simulink model "polyforest2"  (R2024a)
settings: Solver=VariableStepAuto  StartTime=0.0  StopTime=60  RelTol=1e-3
libraries: vrlib x1
settings Model: Creator=samoe  LastModifiedBy=samoe

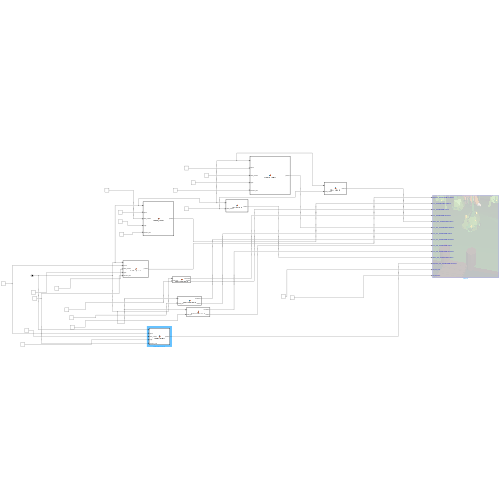
[thumbnail: Simulink's stored preview of the top-level diagram]
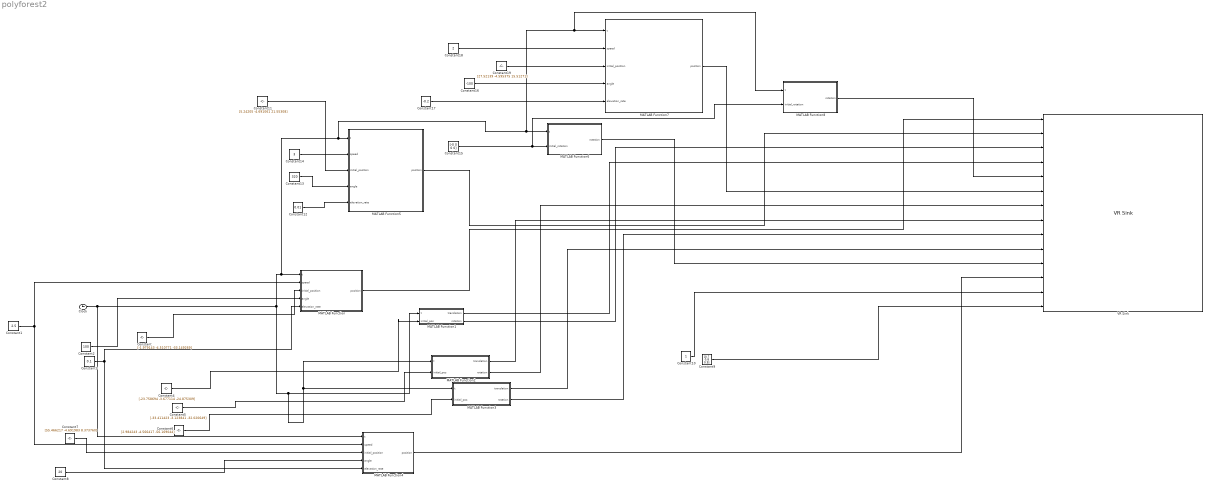
== system polyforest2 ==
  Clock : Clock
  Constant : Constant  Value=[-1.979143 -4.510771 -33.149269]  VectorParams1D=off
  Constant1 : Constant  Value=2.5
  Constant10 : Constant
  Constant11 : Constant  Value=[5.24205 -4.691061 21.55308]  VectorParams1D=off
  Constant12 : Constant  Value=0.01
  Constant13 : Constant  Value=320
  Constant14 : Constant  Value=3
  Constant15 : Constant  Value=[-0 0 0 0]
  Constant16 : Constant  Value=-100
  Constant17 : Constant  Value=-0.2
  Constant18 : Constant  Value=2
  Constant19 : Constant  Value=[27.52139 -4.595375 15.51271]  VectorParams1D=off
  Constant2 : Constant  Value=100
  Constant3 : Constant  Value=0.1
  Constant4 : Constant  Value=[-23.758694 -3.677114 -24.875309]  VectorParams1D=off
  Constant5 : Constant  Value=[-33.411423 -3.123841 -32.020649]  VectorParams1D=off
  Constant6 : Constant  Value=[2.984243 -4.566417 -56.169044]  VectorParams1D=off
  Constant7 : Constant  Value=[55.466217 -4.691983 8.373760]  VectorParams1D=off
  Constant8 : Constant  Value=20
  Constant9 : Constant  Value=[0.7 0.8 0.9]  VectorParams1D=off
  MATLAB Function : MATLAB Function  TreatAsAtomicUnit=on
  MATLAB Function1 : MATLAB Function  TreatAsAtomicUnit=on
  MATLAB Function2 : MATLAB Function  TreatAsAtomicUnit=on
  MATLAB Function3 : MATLAB Function  TreatAsAtomicUnit=on
  MATLAB Function4 : MATLAB Function  TreatAsAtomicUnit=on
  MATLAB Function5 : MATLAB Function  TreatAsAtomicUnit=on
  MATLAB Function6 : MATLAB Function  TreatAsAtomicUnit=on
  MATLAB Function7 : MATLAB Function  TreatAsAtomicUnit=on
  MATLAB Function8 : MATLAB Function  TreatAsAtomicUnit=on
  VR Sink : vrlib/VR Sink  InstantiateOnLoad=on  SampleTime=0.1  ViewEnable=on  RemoteChange=off  RemoteView=off  FieldsWritten=Elephant_TRANSFORM.translation.3.1.1.double#Lion_TRANSFORM.translation.3.1.1.double#Fox_TRANSFORM.rotation.4.1.1.double#Fox_TRANSFORM.translation.3.1.1.double#Zebra_001_TRANSFORM.rotation.4.1.1.double#Lion_001_TRANSFORM.translation.3.1.1.double#Fox_001_TRANSFORM.rotation.4.1.1.double#Fox_001_TRANSFORM.translation.3.1.1.double#Fox_002_TRANSFORM.rotation.4.1.1.double#Fox_002_TRANSFORM.translation.3.1.1.double#Zebra_002_TRANSFORM.rotation.4.1.1.double#Elephant_002_TRANSFORM.translation.3.1.1.double#sky.set_bind.1.1.1.logical#sky.skyColor.3.-1.1.double  WorldFileName=D:\Documents\MATLAB\6.LAST\polyforest.x3d  AutoView=off  VideoDimensions=[]  AllowVariableSize=off
  wires:
  Clock/1 -> MATLAB Function4/1(t), MATLAB Function3/1(t), MATLAB Function2/1(t), MATLAB Function1/1(t), MATLAB Function8/1(t), MATLAB Function7/1(t), MATLAB Function6/1(t), MATLAB Function5/1(t), MATLAB Function/1(t)
  Constant/1 -> MATLAB Function/3(initial_position)
  Constant2/1 -> MATLAB Function/4(angle)
  Constant3/1 -> MATLAB Function4/5(elevation_rate), MATLAB Function/5(elevation_rate)
  Constant4/1 -> MATLAB Function1/2(initial_pos)
  Constant5/1 -> MATLAB Function2/2(initial_pos)
  Constant6/1 -> MATLAB Function3/2(initial_pos)
  Constant7/1 -> MATLAB Function4/3(initial_position)
  Constant1/1 -> MATLAB Function4/2(speed), MATLAB Function/2(speed)
  Constant8/1 -> MATLAB Function4/4(angle)
  Constant11/1 -> MATLAB Function5/3(initial_position)
  Constant14/1 -> MATLAB Function5/2(speed)
  Constant12/1 -> MATLAB Function5/5(elevation_rate)
  Constant13/1 -> MATLAB Function5/4(angle)
  Constant15/1 -> MATLAB Function8/2(initial_rotation), MATLAB Function6/2(initial_rotation)
  MATLAB Function/1(position) -> VR Sink/1
  MATLAB Function5/1(position) -> VR Sink/2
  MATLAB Function1/2(rotation) -> VR Sink/3
  MATLAB Function1/1(translation) -> VR Sink/4
  MATLAB Function2/2(rotation) -> VR Sink/7
  MATLAB Function2/1(translation) -> VR Sink/8
  MATLAB Function3/2(rotation) -> VR Sink/9
  MATLAB Function3/1(translation) -> VR Sink/10
  MATLAB Function4/1(position) -> VR Sink/12
  Constant10/1 -> VR Sink/13
  Constant9/1 -> VR Sink/14
  MATLAB Function6/1(rotation) -> VR Sink/11
  MATLAB Function7/1(position) -> VR Sink/6
  Constant18/1 -> MATLAB Function7/2(speed)
  Constant17/1 -> MATLAB Function7/5(elevation_rate)
  Constant16/1 -> MATLAB Function7/4(angle)
  Constant19/1 -> MATLAB Function7/3(initial_position)
  MATLAB Function8/1(rotation) -> VR Sink/5

== matlab function polyforest2/MATLAB Function1 ==
  data: t input; translation output; rotation output; initial_pos input
function [translation, rotation] = foxRandomMovement(t, initial_pos)
    % foxRandomMovement - Generate a zigzag movement pattern keeping fox on ground
    % 
    % Inputs:
    %   t - Current simulation time
    %   initial_pos - Initial [x, y, z] position of the fox [1x3 matrix]
    %
    % Outputs:
    %   translation - New [x, y, z] position [1x3 matrix]
    %   rotation - Rotation as [x, y, z, angle] [1x4 matrix]
    
    % Movement parameters
    zigzag_width = 1;     % Width of the zigzag path
    forward_speed = -1;    % Forward movement speed
    zigzag_freq = 1;      % Frequency of zigzag motion
    
    % Create zigzag pattern in X-axis (sideways)
    x_move = initial_pos(1) + zigzag_width * sin(zigzag_freq * t);
    
    % Move forward in Z-axis (assuming this is forward direction)
    z_move = initial_pos(3) + forward_speed * t;
    
    % Keep Y-axis (height/vertical) at initial ground level
    y_move = initial_pos(2);
    
    % Create translation vector
    translation = [x_move, y_move, z_move];
    
    % Simple rotation to add some movement interest
    rotation = [0, 1, 0, 0.5 * sin(t)];
end

== matlab function polyforest2/MATLAB Function ==
  data: t input; speed input; initial_position input; position output; angle input; elevation_rate input
function position = translate_forward(t, speed, initial_position, angle, elevation_rate)
% TRANSLATE_FORWARD Calculates the new position of an object moving in a specific direction.
%
% Inputs:
%   t                - Time input from the Simulink clock
%   speed            - Speed of translation (units per second)
%   initial_position - Initial position of the object [x, y, z]
%   angle            - Angle of movement (in radians)
%   elevation_rate   - Rate of increase in the Y-axis (units per second)
%
% Output:
%   position         - Updated position of the object [x, y, z]
    if t<23
        % Compute the displacement magnitude
        displacement = speed * t;
    
        % Calculate the displacement in the X and Z directions
        dx = displacement * cos(angle);
        dz = displacement * sin(angle);
    
        % Calculate the elevation (Y-axis)
        dy = elevation_rate * t; % Increment based on time
    
        % Update the position
       
        position = initial_position + [dx, dy, dz]; % Includes elevation on Y-axis
    else
         % Compute the displacement magnitude
        displacement = speed * 23;
    
        % Calculate the displacement in the X and Z directions
        dx = displacement * cos(angle);
        dz = displacement * sin(angle);
    
        % Calculate the elevation (Y-axis)
        dy = elevation_rate * t; % Increment based on time
    
        % Update the position
       
        position = initial_position + [dx, dy, dz]; % Includes elevation on Y-axis
    end
end

== matlab function polyforest2/MATLAB Function2 ==
  data: t input; translation output; rotation output; initial_pos input
function [translation, rotation] = foxRandomMovement(t, initial_pos)
    % foxRandomMovement - Generate a zigzag movement pattern with randomness
    % 
    % Inputs:
    %   t - Current simulation time
    %   initial_pos - Initial [x, y, z] position of the fox [1x3 matrix]
    %
    % Outputs:
    %   translation - New [x, y, z] position [1x3 matrix]
    %   rotation - Rotation as [x, y, z, angle] [1x4 matrix]
    
    % Movement parameters
    zigzag_width = 5;       % Width of the zigzag path
    forward_speed = -0.5;      % Forward movement speed
    zigzag_freq = 1;        % Frequency of zigzag motion
    random_scale = 0.2;     % Scale for random noise

    % Random noise (scaled)
    random_x = random_scale * randn(); % Sideways randomness
    random_z = random_scale * randn(); % Forward randomness

    % Create zigzag pattern in X-axis (sideways)
    x_move = initial_pos(1) + zigzag_width * sin(zigzag_freq * t) + random_x;

    % Move forward in Z-axis (assuming this is forward direction)
    z_move = initial_pos(3) + forward_speed * t + random_z;

    % Keep Y-axis (height/vertical) at initial ground level
    y_move = initial_pos(2);

    % Create translation vector
    translation = [x_move, y_move, z_move];

    % Add random rotation to simulate natural turning
    random_rotation = 0.1 * randn(); % Small random rotation
    rotation = [0, 1, 0, 0.5 * cos(t) + random_rotation];
end

== matlab function polyforest2/MATLAB Function3 ==
  data: t input; translation output; rotation output; initial_pos input
function [translation, rotation] = foxRandomMovement(t, initial_pos)
    % foxRandomMovement - Generate a zigzag movement pattern with randomness
    % 
    % Inputs:
    %   t - Current simulation time
    %   initial_pos - Initial [x, y, z] position of the fox [1x3 matrix]
    %
    % Outputs:
    %   translation - New [x, y, z] position [1x3 matrix]
    %   rotation - Rotation as [x, y, z, angle] [1x4 matrix]
    
    % Movement parameters
    zigzag_width = 2;       % Width of the zigzag path
    forward_speed = -2;      % Forward movement speed
    zigzag_freq = 0.5;        % Frequency of zigzag motion
    random_scale = 0.5;     % Scale for random noise

    % Random noise (scaled)
    random_x = random_scale * randn(); % Sideways randomness
    random_z = random_scale * randn(); % Forward randomness

    % Create zigzag pattern in X-axis (sideways)
    x_move = initial_pos(1) + zigzag_width * sin(zigzag_freq * t) + random_x;

    % Move forward in Z-axis (assuming this is forward direction)
    z_move = initial_pos(3) + forward_speed * t + random_z;

    % Keep Y-axis (height/vertical) at initial ground level
    y_move = initial_pos(2);

    % Create translation vector
    translation = [x_move, y_move, z_move];

    % Add random rotation to simulate natural turning
    random_rotation = 0.1 * randn(); % Small random rotation
    rotation = [0, 1, 0, 0.5 * cos(t) + random_rotation];
end

== matlab function polyforest2/MATLAB Function4 ==
  data: t input; position output; speed input; initial_position input; angle input; elevation_rate input
function position = translate_forward(t, speed, initial_position, angle, elevation_rate)
% TRANSLATE_FORWARD Calculates the new position of an object moving in a specific direction.
%
% Inputs:
% t - Time input from the Simulink clock
% speed - Speed of translation (units per second)
% initial_position - Initial position of the object [x, y, z]
% angle - Angle of movement (in radians)
% elevation_rate - Rate of increase in the Y-axis (units per second)
%
% Output:
% position - Updated position of the object [x, y, z]

% Check if time is between 44 and 58 seconds
if t >= 44 && t <= 58
    % Compute the displacement magnitude (subtract 44 to start from zero at t=44)
    displacement = speed * (t - 44);
    
    % Calculate the displacement in the X and Z directions
    dx = displacement * cos(angle);
    dz = displacement * sin(angle);
    
    % Calculate the elevation (Y-axis), also starting from t=44
    dy = elevation_rate * (t - 44);
    
    % Update the position
    position = initial_position - [dx, dy, dz]; % Includes elevation on Y-axis
elseif t > 54
    % After t=58, calculate and hold the final position
    displacement = speed * (58 - 44);
    dx = displacement * cos(angle);
    dz = displacement * sin(angle);
    dy = elevation_rate * (58 - 44);
    
    % Hold the final position
    position = initial_position - [dx, dy, dz];
else
    % Before t=44, return the initial position
    position = initial_position;
end
end

== matlab function polyforest2/MATLAB Function5 ==
  data: t input; position output; speed input; initial_position input; angle input; elevation_rate input
function position = translate_forward(t, speed, initial_position, angle, elevation_rate)
% TRANSLATE_FORWARD Calculates the new position of an object moving in a specific direction.
%
% Inputs:
%   t                - Time input from the Simulink clock
%   speed            - Speed of translation (units per second)
%   initial_position - Initial position of the object [x, y, z]
%   angle            - Angle of movement (in degrees)
%   elevation_rate   - Rate of increase in the Y-axis (units per second)
%
% Output:
%   position         - Updated position of the object [x, y, z]

    % Convert angle from degrees to radians
    angle_rad = deg2rad(angle);
    
    % Check if time is less than 23 seconds
    if t < 15
        % Compute the displacement magnitude
        displacement = speed * t;

        % Calculate the displacement in the X and Z directions
        dx = displacement * cos(angle_rad);
        dz = displacement * sin(angle_rad);

        % Calculate the elevation (Y-axis)
        dy = elevation_rate * t; % Increment based on time

        % Update the position
        position = initial_position - [dx, dy, dz]; % Includes elevation on Y-axis
    else
        % Compute the displacement magnitude for the capped time
        displacement = speed * 15;

        % Calculate the displacement in the X and Z directions
        dx = displacement * cos(angle_rad);
        dz = displacement * sin(angle_rad);

        % Calculate the elevation (Y-axis)
        dy = elevation_rate * t; % Increment based on time

        % Update the position
        position = initial_position - [dx, dy, dz]; % Includes elevation on Y-axis
    end
end

== matlab function polyforest2/MATLAB Function6 ==
  data: t input; rotation output; initial_rotation input
function rotation = rotate_about_z(t, initial_rotation)
% ROTATE_ABOUT_Z Rotates an object about the z-axis to simulate a zebra falling, 
% maintaining the final position after a specific time.
%
% Inputs:
% t - Current simulation time
% initial_rotation - Initial rotation as [x, y, z, angle] (1x4 vector)
%
% Output:
% rotation - Updated rotation as [x, y, z, angle] (1x4 vector)

% Ensure rotation is always a 1x4 vector with the same size as initial_rotation
rotation = zeros(size(initial_rotation));
rotation(1:3) = initial_rotation(1:3);

% Compute rotation only within the time range
if t >= 15 && t <= 16
    % Compute rotation angle (proportional to time elapsed)
    % Rotate from 0 to pi (180 degrees) during the 3-second interval
    angle = (t - 15) * pi; % Rotates from 0 to pi over 3 seconds
    
    % Update rotation about the z-axis
    rotation(1) = 0;
    rotation(2) = 0;
    rotation(3) = 1;  % Rotating about z-axis
    rotation(4) = angle;
elseif t > 16
    % After time 18, maintain the final rotated position
    rotation(1) = 0;
    rotation(2) = 0;
    rotation(3) = 1;  % Still z-axis
    rotation(4) = pi/2;  % Fully rotated (180 degrees)
else
    % Retain the original rotation when before rotation time
    rotation = initial_rotation;
end
end

== matlab function polyforest2/MATLAB Function7 ==
  data: t input; position output; speed input; initial_position input; angle input; elevation_rate input
function position = translate_forward(t, speed, initial_position, angle, elevation_rate)
% TRANSLATE_FORWARD Calculates the new position of an object moving in a specific direction.
%
% Inputs:
% t - Time input from the Simulink clock
% speed - Speed of translation (units per second)
% initial_position - Initial position of the object [x, y, z]
% angle - Angle of movement (in degrees)
% elevation_rate - Rate of increase in the Y-axis (units per second)
%
% Output:
% position - Updated position of the object [x, y, z]

% Convert angle from degrees to radians
angle_rad = deg2rad(angle);

% Check if time is 20 seconds or greater, but less than 43
if t >= 20 && t < 43
    % Compute the displacement magnitude (subtract 20 to start from zero at t=20)
    displacement = speed * (t - 20);
    
    % Calculate the displacement in the X and Z directions
    dx = displacement * cos(angle_rad);
    dz = displacement * sin(angle_rad);
    
    % Calculate the elevation (Y-axis), also starting from t=20
    dy = elevation_rate * (t - 20);
    
    % Update the position
    position = initial_position - [dx, dy, dz]; % Includes elevation on Y-axis
elseif t >= 43
    % At t=43 and beyond, calculate the final position and hold it
    displacement = speed * (43 - 20);
    dx = displacement * cos(angle_rad);
    dz = displacement * sin(angle_rad);
    dy = elevation_rate * (43 - 20);
    
    % Hold the position at t=43
    position = initial_position - [dx, dy, dz];
else
    % Before t=20, return the initial position
    position = initial_position;
end
end

== matlab function polyforest2/MATLAB Function8 ==
  data: t input; rotation output; initial_rotation input
function rotation = rotate_about_z(t, initial_rotation)
% ROTATE_ABOUT_Z Rotates an object about the z-axis to simulate a zebra falling, 
% maintaining the final position after a specific time.
%
% Inputs:
% t - Current simulation time
% initial_rotation - Initial rotation as [x, y, z, angle] (1x4 vector)
%
% Output:
% rotation - Updated rotation as [x, y, z, angle] (1x4 vector)

% Ensure rotation is always a 1x4 vector with the same size as initial_rotation
rotation = zeros(size(initial_rotation));
rotation(1:3) = initial_rotation(1:3);

% Compute rotation only within the time range
if t >= 42 && t <= 43
    % Compute rotation angle (proportional to time elapsed)
    % Rotate from 0 to pi (180 degrees) during the 3-second interval
    angle = (t - 15) * pi; % Rotates from 0 to pi over 3 seconds
    
    % Update rotation about the z-axis
    rotation(1) = 0;
    rotation(2) = 0;
    rotation(3) = 1;  % Rotating about z-axis
    rotation(4) = angle;
elseif t > 43
    % After time 18, maintain the final rotated position
    rotation(1) = 0;
    rotation(2) = 0;
    rotation(3) = 1;  % Still z-axis
    rotation(4) = pi/2;  % Fully rotated (180 degrees)
else
    % Retain the original rotation when before rotation time
    rotation = initial_rotation;
end
end
